simulink model "DemonstratorSimscape_GMM1"  (R2021b)
settings: Solver=ode113  StartTime=0.0  StopTime=t_stop*0+20  FixedStep=1e-4
values from neighbouring files (symbols this model uses):
  brkD = 0    [main.m]
  brkI = 1e4    (= 10000)    [main.m]
  brkP = 1e5    (= 100000)    [main.m]
  d_drm = 0.5*d_drum    [main.m]
  d_shm = 0.4*d_sheave    [main.m]
  DeltaCable0 = 0    [main.m]
  Droop_scaling = 0    [main.m]
  eta_sh = 0.015    [main.m]
  filt_NUM = ones(1,200)*0.005    [main.m]
  g = 9.80665    [main.m]
  Iw = 0.5*(W.i + M.in*GB.r^2)    [main.m]
  Kp_mul = 0.3    [main.m]
  Lc0 = abs((T.ph-L.height-P.d-L.z0)*0.001)    [main.m]
  Ls1 = ((T.ph-0.5*W.pd)/1000)    [main.m]
  Ls2 = ((0.5*(T.s2+P.d)-2*P.d)/1000)    [main.m]
  M = 50e3    (= 50000)    [calcGrav.m]
  phi0_drm = -90    [main.m]
  phi0_shm = -90    [main.m]
  r_sheave = P.d*0.5    [main.m]
  s = tf('s')    [calcGrav.m]
  tau_brk = 0.001    [main.m]
  tau_em = 60e-3    (= 0.06)    [calcGrav.m]    (also in main.m)
  tau_m = tau_w/GB.r    [main.m]
  Tmax = 400e3    (= 400000)    [main.m]
  Tn_mul = 10    [main.m]
  x_drm = 0.7*r_drum    [main.m]
  x_shm = 0.7*r_sheave    [main.m]
  z0 = 0    [calcGrav.m]    (also in main.m = L.z0-P.d*0.5-P.d-P.d-L.height-T.h1-T.h2-32)
undefined symbols (not defined in the file or in its folder): C, CA, Controller_sampleTime, DiscIntNeverNeededParam, GB, L, P, Part, T, VFD_acceleration_model_factor, VFD_Adapt_factor_lower_p1458, VFD_Adapt_factor_upper_p1459, VFD_Curr_limit_var_p0641, VFD_Current_limit_p0640, VFD_Id_setp_total_r1624, VFD_Iq, VFD_Kp_n_basic_p1460, VFD_M, VFD_M_accel_T_smooth_p1517, VFD_M_lim_var_fixS_src_p1551, VFD_M_max_lower_p1521, VFD_M_max_lower_scal_p1525, VFD_M_max_up_mot_scal_p1524, VFD_M_max_upper_p1520, VFD_n_act_T_smooth_p1442, VFD_n_ctr_Kp_n_up_scal_p1461, VFD_n_ctr_Tn_n_up_sca_p1463, VFD_n_ctrl_adapt_Kp_lower_p1456, VFD_n_ctrl_adapt_Kp_upper_p1457, VFD_n_ctrl_Adpt_sig_Kp_p1455, VFD_n_ctrl_Kp_scal_p1466, VFD_n_ctrl_n_lower_p1464, VFD_n_ctrl_n_upper_p1465, VFD_n_ctrl_Tn_n_lower_p1462, VFD_n_limit_neg_p1086, VFD_n_limit_pos_p1083, VFD_n_limit_setp_p1063, VFD_n_max_p1082, VFD_n_set_filt_1_T_p1416, VFD_P_max_gen_p1531, VFD_P_max_mot_p1530, VFD_PU_I_outp_max_r0289, VFD_RFG_ramp_down_time_p1121, VFD_RFG_ramp_up_time_p1120, VFD_RFG_t_RD_scal_p1139, VFD_RFG_t_RU_scal_p1138, VSD, W, X, Y, Z
libraries: sm_lib x248, nesl_utility x128, simulink x49, cstblocks x2, pid_lib x2, slpidlib x2, simulink_extras x2
(part 4 of 11)

== system DemonstratorSimscape_GMM1/EM System/Motor Winch Right/Gearbox ==
  MotTrq : Inport
  MotSpd : Inport  Port=2
  GearBox : Gain  Gain=GB.r
  Gearbox efficiency : Subsystem
  Sheaves efficiency : Subsystem
  WinchTrq : Outport
  WinchTrq' : Outport  Port=2
  wires:
  Gearbox efficiency/1(WinchTrq) -> GearBox/1
  MotTrq/1 -> Gearbox efficiency/1(MotTrqRef)
  MotSpd/1 -> Sheaves efficiency/2(MotSpd), Gearbox efficiency/2(MotSpd)
  GearBox/1 -> WinchTrq/1, Sheaves efficiency/1(WinchTrq)
  Sheaves efficiency/1(WinchTrq') -> WinchTrq'/1

== system DemonstratorSimscape_GMM1/EM System/Motor Winch Right/Motor ==
  MotTrqRef : Inport
  MotSpd : Inport  Port=2
  Ideal motor : Subsystem  Commented=on
  Motor dynamics : Subsystem
  Motor with efficiency : Subsystem
  MotTrq : Outport
  wires:
  MotTrqRef/1 -> Motor with efficiency/1(MotTrqRef), Ideal motor/1(MotTrqRef)
  MotSpd/1 -> Motor with efficiency/2(MotSpd)
  Motor dynamics/1(TrqOut) -> MotTrq/1
  Motor with efficiency/1(MotTrq) -> Motor dynamics/1(TrqIn)

== system DemonstratorSimscape_GMM1/EM System/Motor Winch Right/PS>Sim ==
  Gain{1..4} (4 alike) : Gain
  b (rad/s) : nesl_utility/PS-Simulink Converter  PhysicalDomain=network_engine_domain  SubClassName=ps_output  LeftPortType=input  RightPortType=output  PseudoPeriodic=off  Frequencies=[]  Unit=rad/s  AffineConversion=off
      settings: SourceProductBaseCode=PW,SS
  b (rad/s^2) : nesl_utility/PS-Simulink Converter  PhysicalDomain=network_engine_domain  SubClassName=ps_output  LeftPortType=input  RightPortType=output  PseudoPeriodic=off  Frequencies=[]  Unit=rad/s^2  AffineConversion=off
      settings: SourceProductBaseCode=PW,SS
  fc (N) : nesl_utility/PS-Simulink Converter  PhysicalDomain=network_engine_domain  SubClassName=ps_output  LeftPortType=input  RightPortType=output  PseudoPeriodic=off  Frequencies=[]  Unit=N  AffineConversion=off
      settings: SourceProductBaseCode=PW,SS
  ft (N) : nesl_utility/PS-Simulink Converter  PhysicalDomain=network_engine_domain  SubClassName=ps_output  LeftPortType=input  RightPortType=output  PseudoPeriodic=off  Frequencies=[]  Unit=N  AffineConversion=off
      settings: SourceProductBaseCode=PW,SS
  q (deg) : nesl_utility/PS-Simulink Converter  PhysicalDomain=network_engine_domain  SubClassName=ps_output  LeftPortType=input  RightPortType=output  PseudoPeriodic=off  Frequencies=[]  Unit=deg  AffineConversion=off
      settings: SourceProductBaseCode=PW,SS
  t (Nm) : nesl_utility/PS-Simulink Converter  PhysicalDomain=network_engine_domain  SubClassName=ps_output  LeftPortType=input  RightPortType=output  PseudoPeriodic=off  Frequencies=[]  Unit=N*m  AffineConversion=off
      settings: SourceProductBaseCode=PW,SS
  tc (Nm) : nesl_utility/PS-Simulink Converter  PhysicalDomain=network_engine_domain  SubClassName=ps_output  LeftPortType=input  RightPortType=output  PseudoPeriodic=off  Frequencies=[]  Unit=N*m  AffineConversion=off
      settings: SourceProductBaseCode=PW,SS
  tt (Nm) : nesl_utility/PS-Simulink Converter  PhysicalDomain=network_engine_domain  SubClassName=ps_output  LeftPortType=input  RightPortType=output  PseudoPeriodic=off  Frequencies=[]  Unit=N*m  AffineConversion=off
      settings: SourceProductBaseCode=PW,SS
  w (rpm) : nesl_utility/PS-Simulink Converter  PhysicalDomain=network_engine_domain  SubClassName=ps_output  LeftPortType=input  RightPortType=output  PseudoPeriodic=off  Frequencies=[]  Unit=rpm  AffineConversion=off
      settings: SourceProductBaseCode=PW,SS
  q : PMIOPort  Side=Left
  Conn2 : PMIOPort  Port=2  Side=Left
  Conn3 : PMIOPort  Port=3  Side=Left
  Conn4 : PMIOPort  Port=4  Side=Left
  Conn5 : PMIOPort  Port=5  Side=Left
  Conn6 : PMIOPort  Port=6  Side=Left
  Conn7 : PMIOPort  Port=7  Side=Left
  Conn8 : PMIOPort  Port=8  Side=Left
  Out1 : Outport  VectorParamsAs1DForOutWhenUnconnected=off
  Out2 : Outport  Port=2  VectorParamsAs1DForOutWhenUnconnected=off
  Out3 : Outport  Port=3  VectorParamsAs1DForOutWhenUnconnected=off
  Out4 : Outport  Port=4  VectorParamsAs1DForOutWhenUnconnected=off
  Out5 : Outport  Port=5  VectorParamsAs1DForOutWhenUnconnected=off
  Out6 : Outport  Port=6  VectorParamsAs1DForOutWhenUnconnected=off
  Out7 : Outport  Port=7  VectorParamsAs1DForOutWhenUnconnected=off
  Out8 : Outport  Port=8  VectorParamsAs1DForOutWhenUnconnected=off
  Out9 : Outport  Port=9  VectorParamsAs1DForOutWhenUnconnected=off
  wires:
  q (deg)/1 -> Gain1/1
  w (rpm)/1 -> Gain2/1
  b (rad/s^2)/1 -> Gain3/1
  t (Nm)/1 -> Gain4/1
  fc (N)/1 -> Out5/1
  tc (Nm)/1 -> Out6/1
  ft (N)/1 -> Out7/1
  tt (Nm)/1 -> Out8/1
  Gain1/1 -> Out1/1
  Gain2/1 -> Out2/1
  Gain3/1 -> Out3/1
  Gain4/1 -> Out4/1
  b (rad/s)/1 -> Out9/1
  connections:
  q/RConn1 -- q (deg)/LConn1
  Conn2/RConn1 -- b (rad/s)/LConn1 -- w (rpm)/LConn1
  Conn3/RConn1 -- b (rad/s^2)/LConn1
  Conn4/RConn1 -- t (Nm)/LConn1
  fc (N)/LConn1 -- Conn5/RConn1
  Conn6/RConn1 -- tc (Nm)/LConn1
  ft (N)/LConn1 -- Conn7/RConn1
  Conn8/RConn1 -- tt (Nm)/LConn1

== system DemonstratorSimscape_GMM1/EM System/Winch Left (yellow)/Variable Winch Inertia ==
  WinchAngle (deg) : Inport
  Constant : Constant  Value=W.d/2
  Demux : Demux  Outputs=3
  Gain1 : Gain  Gain=-1
  Gain2 : Gain  Gain=0.5
  S-Function : S-Function  FunctionName=sfun_wcable  Parameters=W.n0,W.perc0,W.dpl,W.alpha_r,CA.mpl,W.d,CA.d  SFunctionDeploymentMode=off  EnableBusSupport=off
  Simulink-PS Converter : nesl_utility/Simulink-PS Converter  PhysicalDomain=network_engine_domain  SubClassName=ps_input  LeftPortType=input  RightPortType=output  PseudoPeriodic=off  Frequencies=[]  NoiseDistribution=none  NoiseParameters=[]  Unit=kg  AffineConversion=on  FilteringAndDerivatives=zero  SimscapeFilterOrder=2  InputFilterTimeConstant=0.001  UdotUserProvided=0
      settings: SourceProductBaseCode=PW,SS
  WinchCable : Scope  Commented=on  NumInputPorts=4
  cable on Winch Variable Mass : sm_lib/Body Elements/Variable Mass/General Variable Mass  VariableInertiaType=PointMass  MassType=TimeVarying  Mass=1  MassUnits=kg  CenterOfMassType=Constant  CenterOfMass=[0 0 0]  CenterOfMassUnits=m  InertiaMatrixType=Constant  MomentsOfInertia=[1 1 1]  MomentsOfInertiaUnits=kg*m^2  ProductsOfInertia=[0 0 0]  ProductsOfInertiaUnits=kg*m^2  GraphicType=None  MarkerShape=Sphere  MarkerSize=10  GraphicVisPropType=SimpleVisualProperties  GraphicDiffuseColor=[0.5 0.5 0.5]  GraphicSpecularColor=[0.5 0.5 0.5 1.0]  GraphicAmbientColor=[0.15 0.15 0.15 1.0]  GraphicEmissiveColor=[0.0 0.0 0.0 1.0]  GraphicShininess=75  GraphicOpacity=1.0
      settings: SourceProductBaseCode=MS
  CableInertia : PMIOPort  Side=Right
  CableLayer : Outport
  WinchRadius (mm) : Outport  Port=2  VectorParamsAs1DForOutWhenUnconnected=off
  wires:
  Demux/1 -> WinchCable/3, Simulink-PS Converter/1
  Gain1/1 -> S-Function/1
  S-Function/1 -> Demux/1
  Demux/2 -> WinchCable/1, CableLayer/1
  WinchAngle (deg)/1 -> Gain1/1
  Demux/3 -> WinchRadius (mm)/1
  [CableMass] -> Gain2/1
  Gain2/1 -> WinchCable/4
  Constant/1 -> WinchCable/2
  connections:
  cable on Winch Variable Mass/RConn1 -- CableInertia/RConn1
  Simulink-PS Converter/RConn1 -- cable on Winch Variable Mass/LConn1

== system DemonstratorSimscape_GMM1/EM System/Winch Left (yellow)/tags ==
  Rigid Transform1 : sm_lib/Frames and Transforms/Rigid Transform  TranslationMethod=Cartesian  TranslationStandardOffset=0  TranslationLengthUnit=mm  TranslationStandardAxis=+Z  TranslationCartesianOffset=[x_drm*cosd(phi0+120), x_drm*sind(phi0+120), s*d_drm]  TranslationROffset=0  TranslationROffsetUnits=m  TranslationZOffset=0  TranslationZOffsetUnits=m  TranslationThetaOffset=0  TranslationThetaOffsetUnits=deg  RotationMethod=None  RotationAngleUnits=deg  RotationStandardAxis=+Z  RotationAngle=0.0  RotationArbitraryAxis=[0 0 1]  FollAlignAxisA=+X  BaseAlignAxisA=+Y  FollAlignAxisB=+Y  BaseAlignAxisB=+Z  RotationSequenceAxes=FollowerAxes  RotationSequence=XYX  RotationSequenceAngles=[0 0 0]  RotationSequenceAnglesUnits=deg  RotationMatrix=[1 0 0; 0 1 0; 0 0 1]
  Rigid Transform2 : sm_lib/Frames and Transforms/Rigid Transform  TranslationMethod=Cartesian  TranslationStandardOffset=0  TranslationLengthUnit=mm  TranslationStandardAxis=+Z  TranslationCartesianOffset=[x_drm*cosd(phi0+0), x_drm*sind(phi0+0), s*d_drm]  TranslationROffset=0  TranslationROffsetUnits=m  TranslationZOffset=0  TranslationZOffsetUnits=m  TranslationThetaOffset=0  TranslationThetaOffsetUnits=deg  RotationMethod=None  RotationAngleUnits=deg  RotationStandardAxis=+Z  RotationAngle=0.0  RotationArbitraryAxis=[0 0 1]  FollAlignAxisA=+X  BaseAlignAxisA=+Y  FollAlignAxisB=+Y  BaseAlignAxisB=+Z  RotationSequenceAxes=FollowerAxes  RotationSequence=XYX  RotationSequenceAngles=[0 0 0]  RotationSequenceAnglesUnits=deg  RotationMatrix=[1 0 0; 0 1 0; 0 0 1]
  Rigid Transform3 : sm_lib/Frames and Transforms/Rigid Transform  TranslationMethod=Cartesian  TranslationStandardOffset=0  TranslationLengthUnit=mm  TranslationStandardAxis=+Z  TranslationCartesianOffset=[x_drm*cosd(phi0-120), x_drm*sind(phi0-120), s*d_drm]  TranslationROffset=0  TranslationROffsetUnits=m  TranslationZOffset=0  TranslationZOffsetUnits=m  TranslationThetaOffset=0  TranslationThetaOffsetUnits=deg  RotationMethod=None  RotationAngleUnits=deg  RotationStandardAxis=+Z  RotationAngle=0.0  RotationArbitraryAxis=[0 0 1]  FollAlignAxisA=+X  BaseAlignAxisA=+Y  FollAlignAxisB=+Y  BaseAlignAxisB=+Z  RotationSequenceAxes=FollowerAxes  RotationSequence=XYX  RotationSequenceAngles=[0 0 0]  RotationSequenceAnglesUnits=deg  RotationMatrix=[1 0 0; 0 1 0; 0 0 1]
  tag1 : sm_lib/Body Elements/Cylindrical Solid  GraphicAmbientColor=[0.15 0.15 0.15 1.0]  BasedOnType=Density  CenterOfMass=[0 0 0]  CenterOfMassUnits=m  GraphicDiffuseColor=c_shm  CylinderLength=d_drm  CylinderLengthUnits=mm  CylinderRadius=r_drm  CylinderRadiusUnits=mm  Density=0  DensityUnits=kg/m^3  DoExposeReferenceFrame=on  GraphicEmissiveColor=[0.0 0.0 0.0 1.0]  ExportEntireGeometry=off  SerializedFrames=<Frames/>  MarkerShape=Frame  MarkerSize=10  GraphicType=FromGeometry  InertiaType=CalculateFromGeometry  Mass=0  MassUnits=kg  MomentsOfInertia=[1 1 1]  MomentsOfInertiaUnits=kg*m^2  GraphicOpacity=1.0  ProductsOfInertia=[0 0 0]  ProductsOfInertiaUnits=kg*m^2  GraphicShininess=10  GraphicSpecularColor=[0.8 0.8 0.8]  GraphicVisPropType=SimpleVisualProperties
  tag2 : sm_lib/Body Elements/Cylindrical Solid  GraphicAmbientColor=[0.15 0.15 0.15 1.0]  BasedOnType=Density  CenterOfMass=[0 0 0]  CenterOfMassUnits=m  GraphicDiffuseColor=c_shm  CylinderLength=d_drm  CylinderLengthUnits=mm  CylinderRadius=r_drm  CylinderRadiusUnits=mm  Density=0  DensityUnits=kg/m^3  DoExposeReferenceFrame=on  GraphicEmissiveColor=[0.0 0.0 0.0 1.0]  ExportEntireGeometry=off  SerializedFrames=<Frames/>  MarkerShape=Frame  MarkerSize=10  GraphicType=FromGeometry  InertiaType=CalculateFromGeometry  Mass=0  MassUnits=kg  MomentsOfInertia=[1 1 1]  MomentsOfInertiaUnits=kg*m^2  GraphicOpacity=1.0  ProductsOfInertia=[0 0 0]  ProductsOfInertiaUnits=kg*m^2  GraphicShininess=10  GraphicSpecularColor=[0.8 0.8 0.8]  GraphicVisPropType=SimpleVisualProperties
  tag3 : sm_lib/Body Elements/Cylindrical Solid  GraphicAmbientColor=[0.15 0.15 0.15 1.0]  BasedOnType=Density  CenterOfMass=[0 0 0]  CenterOfMassUnits=m  GraphicDiffuseColor=c_shm  CylinderLength=d_drm  CylinderLengthUnits=mm  CylinderRadius=r_drm  CylinderRadiusUnits=mm  Density=0  DensityUnits=kg/m^3  DoExposeReferenceFrame=on  GraphicEmissiveColor=[0.0 0.0 0.0 1.0]  ExportEntireGeometry=off  SerializedFrames=<Frames/>  MarkerShape=Frame  MarkerSize=10  GraphicType=FromGeometry  InertiaType=CalculateFromGeometry  Mass=0  MassUnits=kg  MomentsOfInertia=[1 1 1]  MomentsOfInertiaUnits=kg*m^2  GraphicOpacity=1.0  ProductsOfInertia=[0 0 0]  ProductsOfInertiaUnits=kg*m^2  GraphicShininess=10  GraphicSpecularColor=[0.8 0.8 0.8]  GraphicVisPropType=SimpleVisualProperties
  Conn1 : PMIOPort  Side=Left
  connections:
  tag2/RConn1 -- Rigid Transform1/RConn1
  Conn1/RConn1 -- Rigid Transform2/LConn1 -- Rigid Transform1/LConn1 -- Rigid Transform3/LConn1
  Rigid Transform2/RConn1 -- tag1/RConn1
  tag3/RConn1 -- Rigid Transform3/RConn1

== system DemonstratorSimscape_GMM1/EM System/Winch Right (blue)/Variable Winch Inertia ==
  WinchAngle (deg) : Inport
  Demux : Demux  Outputs=3
  S-Function : S-Function  FunctionName=sfun_wcable  Parameters=W.n0,W.perc0,W.dpl,W.alpha_r,CA.mpl,W.d,CA.d  SFunctionDeploymentMode=off  EnableBusSupport=off
  Simulink-PS Converter : nesl_utility/Simulink-PS Converter  PhysicalDomain=network_engine_domain  SubClassName=ps_input  LeftPortType=input  RightPortType=output  PseudoPeriodic=off  Frequencies=[]  NoiseDistribution=none  NoiseParameters=[]  Unit=kg  AffineConversion=on  FilteringAndDerivatives=zero  SimscapeFilterOrder=2  InputFilterTimeConstant=0.001  UdotUserProvided=0
      settings: SourceProductBaseCode=PW,SS
  cable on Winch Variable Mass : sm_lib/Body Elements/Variable Mass/General Variable Mass  VariableInertiaType=PointMass  MassType=TimeVarying  Mass=1  MassUnits=kg  CenterOfMassType=Constant  CenterOfMass=[0 0 0]  CenterOfMassUnits=m  InertiaMatrixType=Constant  MomentsOfInertia=[1 1 1]  MomentsOfInertiaUnits=kg*m^2  ProductsOfInertia=[0 0 0]  ProductsOfInertiaUnits=kg*m^2  GraphicType=None  MarkerShape=Sphere  MarkerSize=10  GraphicVisPropType=SimpleVisualProperties  GraphicDiffuseColor=[0.5 0.5 0.5]  GraphicSpecularColor=[0.5 0.5 0.5 1.0]  GraphicAmbientColor=[0.15 0.15 0.15 1.0]  GraphicEmissiveColor=[0.0 0.0 0.0 1.0]  GraphicShininess=75  GraphicOpacity=1.0
      settings: SourceProductBaseCode=MS
  CableInertia : PMIOPort  Side=Right
  CableLayer : Outport
  WinchRadius (mm) : Outport  Port=2  VectorParamsAs1DForOutWhenUnconnected=off
  wires:
  Demux/1 -> Simulink-PS Converter/1
  WinchAngle (deg)/1 -> S-Function/1
  S-Function/1 -> Demux/1
  Demux/2 -> CableLayer/1
  Demux/3 -> WinchRadius (mm)/1
  connections:
  cable on Winch Variable Mass/RConn1 -- CableInertia/RConn1
  Simulink-PS Converter/RConn1 -- cable on Winch Variable Mass/LConn1

== system DemonstratorSimscape_GMM1/EM System/Winch Right (blue)/tags ==
  Rigid Transform1 : sm_lib/Frames and Transforms/Rigid Transform  TranslationMethod=Cartesian  TranslationStandardOffset=0  TranslationLengthUnit=mm  TranslationStandardAxis=+Z  TranslationCartesianOffset=[x_drm*cosd(phi0+120), x_drm*sind(phi0+120), s*d_drm]  TranslationROffset=0  TranslationROffsetUnits=m  TranslationZOffset=0  TranslationZOffsetUnits=m  TranslationThetaOffset=0  TranslationThetaOffsetUnits=deg  RotationMethod=None  RotationAngleUnits=deg  RotationStandardAxis=+Z  RotationAngle=0.0  RotationArbitraryAxis=[0 0 1]  FollAlignAxisA=+X  BaseAlignAxisA=+Y  FollAlignAxisB=+Y  BaseAlignAxisB=+Z  RotationSequenceAxes=FollowerAxes  RotationSequence=XYX  RotationSequenceAngles=[0 0 0]  RotationSequenceAnglesUnits=deg  RotationMatrix=[1 0 0; 0 1 0; 0 0 1]
  Rigid Transform2 : sm_lib/Frames and Transforms/Rigid Transform  TranslationMethod=Cartesian  TranslationStandardOffset=0  TranslationLengthUnit=mm  TranslationStandardAxis=+Z  TranslationCartesianOffset=[x_drm*cosd(phi0+0), x_drm*sind(phi0+0), s*d_drm]  TranslationROffset=0  TranslationROffsetUnits=m  TranslationZOffset=0  TranslationZOffsetUnits=m  TranslationThetaOffset=0  TranslationThetaOffsetUnits=deg  RotationMethod=None  RotationAngleUnits=deg  RotationStandardAxis=+Z  RotationAngle=0.0  RotationArbitraryAxis=[0 0 1]  FollAlignAxisA=+X  BaseAlignAxisA=+Y  FollAlignAxisB=+Y  BaseAlignAxisB=+Z  RotationSequenceAxes=FollowerAxes  RotationSequence=XYX  RotationSequenceAngles=[0 0 0]  RotationSequenceAnglesUnits=deg  RotationMatrix=[1 0 0; 0 1 0; 0 0 1]
  Rigid Transform3 : sm_lib/Frames and Transforms/Rigid Transform  TranslationMethod=Cartesian  TranslationStandardOffset=0  TranslationLengthUnit=mm  TranslationStandardAxis=+Z  TranslationCartesianOffset=[x_drm*cosd(phi0-120), x_drm*sind(phi0-120), s*d_drm]  TranslationROffset=0  TranslationROffsetUnits=m  TranslationZOffset=0  TranslationZOffsetUnits=m  TranslationThetaOffset=0  TranslationThetaOffsetUnits=deg  RotationMethod=None  RotationAngleUnits=deg  RotationStandardAxis=+Z  RotationAngle=0.0  RotationArbitraryAxis=[0 0 1]  FollAlignAxisA=+X  BaseAlignAxisA=+Y  FollAlignAxisB=+Y  BaseAlignAxisB=+Z  RotationSequenceAxes=FollowerAxes  RotationSequence=XYX  RotationSequenceAngles=[0 0 0]  RotationSequenceAnglesUnits=deg  RotationMatrix=[1 0 0; 0 1 0; 0 0 1]
  tag1 : sm_lib/Body Elements/Cylindrical Solid  GraphicAmbientColor=[0.15 0.15 0.15 1.0]  BasedOnType=Density  CenterOfMass=[0 0 0]  CenterOfMassUnits=m  GraphicDiffuseColor=c_shm  CylinderLength=d_drm  CylinderLengthUnits=mm  CylinderRadius=r_drm  CylinderRadiusUnits=mm  Density=0  DensityUnits=kg/m^3  DoExposeReferenceFrame=on  GraphicEmissiveColor=[0.0 0.0 0.0 1.0]  ExportEntireGeometry=off  SerializedFrames=<Frames/>  MarkerShape=Frame  MarkerSize=10  GraphicType=FromGeometry  InertiaType=CalculateFromGeometry  Mass=0  MassUnits=kg  MomentsOfInertia=[1 1 1]  MomentsOfInertiaUnits=kg*m^2  GraphicOpacity=1.0  ProductsOfInertia=[0 0 0]  ProductsOfInertiaUnits=kg*m^2  GraphicShininess=10  GraphicSpecularColor=[0.8 0.8 0.8]  GraphicVisPropType=SimpleVisualProperties
  tag2 : sm_lib/Body Elements/Cylindrical Solid  GraphicAmbientColor=[0.15 0.15 0.15 1.0]  BasedOnType=Density  CenterOfMass=[0 0 0]  CenterOfMassUnits=m  GraphicDiffuseColor=c_shm  CylinderLength=d_drm  CylinderLengthUnits=mm  CylinderRadius=r_drm  CylinderRadiusUnits=mm  Density=0  DensityUnits=kg/m^3  DoExposeReferenceFrame=on  GraphicEmissiveColor=[0.0 0.0 0.0 1.0]  ExportEntireGeometry=off  SerializedFrames=<Frames/>  MarkerShape=Frame  MarkerSize=10  GraphicType=FromGeometry  InertiaType=CalculateFromGeometry  Mass=0  MassUnits=kg  MomentsOfInertia=[1 1 1]  MomentsOfInertiaUnits=kg*m^2  GraphicOpacity=1.0  ProductsOfInertia=[0 0 0]  ProductsOfInertiaUnits=kg*m^2  GraphicShininess=10  GraphicSpecularColor=[0.8 0.8 0.8]  GraphicVisPropType=SimpleVisualProperties
  tag3 : sm_lib/Body Elements/Cylindrical Solid  GraphicAmbientColor=[0.15 0.15 0.15 1.0]  BasedOnType=Density  CenterOfMass=[0 0 0]  CenterOfMassUnits=m  GraphicDiffuseColor=c_shm  CylinderLength=d_drm  CylinderLengthUnits=mm  CylinderRadius=r_drm  CylinderRadiusUnits=mm  Density=0  DensityUnits=kg/m^3  DoExposeReferenceFrame=on  GraphicEmissiveColor=[0.0 0.0 0.0 1.0]  ExportEntireGeometry=off  SerializedFrames=<Frames/>  MarkerShape=Frame  MarkerSize=10  GraphicType=FromGeometry  InertiaType=CalculateFromGeometry  Mass=0  MassUnits=kg  MomentsOfInertia=[1 1 1]  MomentsOfInertiaUnits=kg*m^2  GraphicOpacity=1.0  ProductsOfInertia=[0 0 0]  ProductsOfInertiaUnits=kg*m^2  GraphicShininess=10  GraphicSpecularColor=[0.8 0.8 0.8]  GraphicVisPropType=SimpleVisualProperties
  Conn1 : PMIOPort  Side=Left
  connections:
  tag2/RConn1 -- Rigid Transform1/RConn1
  Conn1/RConn1 -- Rigid Transform2/LConn1 -- Rigid Transform1/LConn1 -- Rigid Transform3/LConn1
  Rigid Transform2/RConn1 -- tag1/RConn1
  tag3/RConn1 -- Rigid Transform3/RConn1

== system DemonstratorSimscape_GMM1/Transmission System/Anchor and Load/CableFlex_Left ==
  disp [m] : Inport
  FlexDisp : Scope  Commented=on  NumInputPorts=4
  Inertia1 : sm_lib/Body Elements/Inertia  InertiaType=PointMass  Mass=0.00000001  MassUnits=kg  CenterOfMass=[0 0 0]  CenterOfMassUnits=m  MomentsOfInertia=[1 1 1]  MomentsOfInertiaUnits=kg*m^2  ProductsOfInertia=[0 0 0]  ProductsOfInertiaUnits=kg*m^2  GraphicType=None  MarkerShape=Inertia  MarkerSize=20  GraphicVisPropType=SimpleVisualProperties  GraphicDiffuseColor=[0.5 0.5 0.5]  GraphicSpecularColor=[0.5 0.5 0.5 1.0]  GraphicAmbientColor=[0.15 0.15 0.15 1.0]  GraphicEmissiveColor=[0.0 0.0 0.0 1.0]  GraphicShininess=75  GraphicOpacity=1.0
  Inertia2 : sm_lib/Body Elements/Inertia  InertiaType=PointMass  Mass=0.00000001  MassUnits=kg  CenterOfMass=[0 0 0]  CenterOfMassUnits=m  MomentsOfInertia=[1 1 1]  MomentsOfInertiaUnits=kg*m^2  ProductsOfInertia=[0 0 0]  ProductsOfInertiaUnits=kg*m^2  GraphicType=None  MarkerShape=Inertia  MarkerSize=20  GraphicVisPropType=SimpleVisualProperties  GraphicDiffuseColor=[0.5 0.5 0.5]  GraphicSpecularColor=[0.5 0.5 0.5 1.0]  GraphicAmbientColor=[0.15 0.15 0.15 1.0]  GraphicEmissiveColor=[0.0 0.0 0.0 1.0]  GraphicShininess=75  GraphicOpacity=1.0
  Mux : Mux  Commented=on  Inputs=2
  Mux1 : Mux  Commented=on  Inputs=2
  PS-Simulink Converter : nesl_utility/PS-Simulink Converter  Commented=on  PhysicalDomain=network_engine_domain  SubClassName=ps_output  LeftPortType=input  RightPortType=output  PseudoPeriodic=off  Frequencies=[]  Unit=m  AffineConversion=off
      settings: SourceProductBaseCode=PW,SS
  PS-Simulink Converter1 : nesl_utility/PS-Simulink Converter  Commented=on  PhysicalDomain=network_engine_domain  SubClassName=ps_output  LeftPortType=input  RightPortType=output  PseudoPeriodic=off  Frequencies=[]  Unit=m/s  AffineConversion=off
      settings: SourceProductBaseCode=PW,SS
  PS-Simulink Converter2 : nesl_utility/PS-Simulink Converter  Commented=on  PhysicalDomain=network_engine_domain  SubClassName=ps_output  LeftPortType=input  RightPortType=output  PseudoPeriodic=off  Frequencies=[]  Unit=m  AffineConversion=off
      settings: SourceProductBaseCode=PW,SS
  PS-Simulink Converter3 : nesl_utility/PS-Simulink Converter  Commented=on  PhysicalDomain=network_engine_domain  SubClassName=ps_output  LeftPortType=input  RightPortType=output  PseudoPeriodic=off  Frequencies=[]  Unit=m/s  AffineConversion=off
      settings: SourceProductBaseCode=PW,SS
  PS-Simulink Converter4 : nesl_utility/PS-Simulink Converter  Commented=on  PhysicalDomain=network_engine_domain  SubClassName=ps_output  LeftPortType=input  RightPortType=output  PseudoPeriodic=off  Frequencies=[]  Unit=m  AffineConversion=off
      settings: SourceProductBaseCode=PW,SS
  PS-Simulink Converter5 : nesl_utility/PS-Simulink Converter  Commented=on  PhysicalDomain=network_engine_domain  SubClassName=ps_output  LeftPortType=input  RightPortType=output  PseudoPeriodic=off  Frequencies=[]  Unit=m/s  AffineConversion=off
      settings: SourceProductBaseCode=PW,SS
  Prismatic Joint : sm_lib/Joints/Prismatic Joint  JointMode=Normal  SenseConstraintForce=off  SenseConstraintForceX=off  SenseConstraintForceY=off  SenseConstraintForceZ=off  SenseConstraintTorque=off  SenseConstraintTorqueX=off  SenseConstraintTorqueY=off  SenseConstraintTorqueZ=off  SenseTotalForce=off  SenseTotalForceX=off  SenseTotalForceY=off  SenseTotalForceZ=off  SenseTotalTorque=off  SenseTotalTorqueX=off  SenseTotalTorqueY=off  SenseTotalTorqueZ=off  CompositeWrenchDir=FollowerOnBase  CompositeWrenchFrame=BaseFrame  EquilibriumPosition=0  EquilibriumPositionUnits=m  SpringStiffness=0  SpringStiffnessUnits=N/m  DampingCoefficient=0  DampingCoefficientUnits=N/(m/s)  TorqueActuationMode=ComputedTorque  MotionActuationMode=InputMotion  SensePosition=off  SenseVelocity=off  SenseAcceleration=off  SenseTorqueForce=off  SenseLowerLimitTorqueForce=off  SenseUpperLimitTorqueForce=off  LowerLimitSpecify=off  LowerLimitBound=-1  LowerLimitBoundUnits=m  LowerLimitStiffness=1e6  LowerLimitStiffnessUnits=N/m  LowerLimitDamping=1e3  LowerLimitDampingUnits=N/(m/s)  LowerLimitTransitionRegionWidth=1e-4  LowerLimitTransitionRegionWidthUnits=m  UpperLimitSpecify=off  UpperLimitBound=1  UpperLimitBoundUnits=m  UpperLimitStiffness=1e6  UpperLimitStiffnessUnits=N/m  UpperLimitDamping=1e3  UpperLimitDampingUnits=N/(m/s)  UpperLimitTransitionRegionWidth=1e-4  UpperLimitTransitionRegionWidthUnits=m  PositionTargetSpecify=on  PositionTargetPriority=High  PositionTargetValue=DeltaCable0*0  PositionTargetValueUnits=mm  VelocityTargetSpecify=off  VelocityTargetPriority=High  VelocityTargetValue=0  VelocityTargetValueUnits=m/s
  Rigid Transform1 : sm_lib/Frames and Transforms/Rigid Transform  TranslationMethod=None  TranslationStandardOffset=0  TranslationLengthUnit=m  TranslationStandardAxis=+Z  TranslationCartesianOffset=[0 0 0]  TranslationROffset=0  TranslationROffsetUnits=m  TranslationZOffset=0  TranslationZOffsetUnits=m  TranslationThetaOffset=0  TranslationThetaOffsetUnits=deg  RotationMethod=StandardAxis  RotationAngleUnits=deg  RotationStandardAxis=+X  RotationAngle=-90  RotationArbitraryAxis=[0 0 1]  FollAlignAxisA=+X  BaseAlignAxisA=+Y  FollAlignAxisB=+Y  BaseAlignAxisB=+Z  RotationSequenceAxes=FollowerAxes  RotationSequence=XYX  RotationSequenceAngles=[0 0 0]  RotationSequenceAnglesUnits=deg  RotationMatrix=[1 0 0; 0 1 0; 0 0 1]
  Rigid Transform2 : sm_lib/Frames and Transforms/Rigid Transform  TranslationMethod=None  TranslationStandardOffset=0  TranslationLengthUnit=m  TranslationStandardAxis=+Z  TranslationCartesianOffset=[0 0 0]  TranslationROffset=0  TranslationROffsetUnits=m  TranslationZOffset=0  TranslationZOffsetUnits=m  TranslationThetaOffset=0  TranslationThetaOffsetUnits=deg  RotationMethod=StandardAxis  RotationAngleUnits=deg  RotationStandardAxis=+X  RotationAngle=90  RotationArbitraryAxis=[0 0 1]  FollAlignAxisA=+X  BaseAlignAxisA=+Y  FollAlignAxisB=+Y  BaseAlignAxisB=+Z  RotationSequenceAxes=FollowerAxes  RotationSequence=XYX  RotationSequenceAngles=[0 0 0]  RotationSequenceAnglesUnits=deg  RotationMatrix=[1 0 0; 0 1 0; 0 0 1]
  Simulink-PS Converter1 : nesl_utility/Simulink-PS Converter  PhysicalDomain=network_engine_domain  SubClassName=ps_input  LeftPortType=input  RightPortType=output  PseudoPeriodic=off  Frequencies=[]  NoiseDistribution=none  NoiseParameters=[]  Unit=m  AffineConversion=on  FilteringAndDerivatives=filter  SimscapeFilterOrder=2  InputFilterTimeConstant=0.001  UdotUserProvided=2
      settings: SourceProductBaseCode=PW,SS
  Transform Sensor : sm_lib/Frames and Transforms/Transform Sensor  Commented=on  MeasurementFrame=World  SenseAngle=off  SenseAxis=off  SenseAngle1=off  SenseAngle2=off  SenseAngle3=off  SenseQ=off  SenseR=off  SenseOmegaX=off  SenseOmegaY=off  SenseOmegaZ=off  SenseOmega1=off  SenseOmega2=off  SenseOmega3=off  SenseQDot=off  SenseRDot=off  SenseAlphaX=off  SenseAlphaY=off  SenseAlphaZ=off  SenseAlpha1=off  SenseAlpha2=off  SenseAlpha3=off  SenseQDDot=off  SenseRDDot=off  SenseX=off  SenseY=on  SenseZ=off  SenseRad=off  SenseAzim=off  SenseDist=off  SenseInc=off  SenseXDot=off  SenseYDot=on  SenseZDot=off  SenseRadDot=off  SenseAzimDot=off  SenseDistDot=off  SenseIncDot=off  SenseXDDot=off  SenseYDDot=off  SenseZDDot=off  SenseRadDDot=off  SenseAzimDDot=off  SenseDistDDot=off  SenseIncDDot=off
  Transform Sensor1 : sm_lib/Frames and Transforms/Transform Sensor  Commented=on  MeasurementFrame=World  SenseAngle=off  SenseAxis=off  SenseAngle1=off  SenseAngle2=off  SenseAngle3=off  SenseQ=off  SenseR=off  SenseOmegaX=off  SenseOmegaY=off  SenseOmegaZ=off  SenseOmega1=off  SenseOmega2=off  SenseOmega3=off  SenseQDot=off  SenseRDot=off  SenseAlphaX=off  SenseAlphaY=off  SenseAlphaZ=off  SenseAlpha1=off  SenseAlpha2=off  SenseAlpha3=off  SenseQDDot=off  SenseRDDot=off  SenseX=off  SenseY=on  SenseZ=off  SenseRad=off  SenseAzim=off  SenseDist=off  SenseInc=off  SenseXDot=off  SenseYDot=on  SenseZDot=off  SenseRadDot=off  SenseAzimDot=off  SenseDistDot=off  SenseIncDot=off  SenseXDDot=off  SenseYDDot=off  SenseZDDot=off  SenseRadDDot=off  SenseAzimDDot=off  SenseDistDDot=off  SenseIncDDot=off
  Transform Sensor2 : sm_lib/Frames and Transforms/Transform Sensor  Commented=on  MeasurementFrame=World  SenseAngle=off  SenseAxis=off  SenseAngle1=off  SenseAngle2=off  SenseAngle3=off  SenseQ=off  SenseR=off  SenseOmegaX=off  SenseOmegaY=off  SenseOmegaZ=off  SenseOmega1=off  SenseOmega2=off  SenseOmega3=off  SenseQDot=off  SenseRDot=off  SenseAlphaX=off  SenseAlphaY=off  SenseAlphaZ=off  SenseAlpha1=off  SenseAlpha2=off  SenseAlpha3=off  SenseQDDot=off  SenseRDDot=off  SenseX=off  SenseY=on  SenseZ=off  SenseRad=off  SenseAzim=off  SenseDist=off  SenseInc=off  SenseXDot=off  SenseYDot=on  SenseZDot=off  SenseRadDot=off  SenseAzimDot=off  SenseDistDot=off  SenseIncDot=off  SenseXDDot=off  SenseYDDot=off  SenseZDDot=off  SenseRadDDot=off  SenseAzimDDot=off  SenseDistDDot=off  SenseIncDDot=off
  World Frame : sm_lib/Frames and Transforms/World Frame  Commented=on
  F : PMIOPort  Side=Right
  B : PMIOPort  Port=2  Side=Left
  wires:
  disp [m]/1 -> Simulink-PS Converter1/1
  Mux/1 -> FlexDisp/1
  Mux1/1 -> FlexDisp/3
  PS-Simulink Converter4/1 -> FlexDisp/2
  PS-Simulink Converter5/1 -> FlexDisp/4
  PS-Simulink Converter/1 -> Mux/1
  PS-Simulink Converter1/1 -> Mux1/1
  PS-Simulink Converter2/1 -> Mux/2
  PS-Simulink Converter3/1 -> Mux1/2
  connections:
  B/RConn1 -- Transform Sensor2/LConn1 -- Transform Sensor/RConn1 -- Rigid Transform2/LConn1
  Simulink-PS Converter1/RConn1 -- Prismatic Joint/LConn2
  Inertia2/RConn1 -- Prismatic Joint/LConn1 -- Rigid Transform1/LConn1
  Inertia1/RConn1 -- Prismatic Joint/RConn1 -- Rigid Transform2/RConn1
  F/RConn1 -- Transform Sensor2/RConn1 -- Transform Sensor1/RConn1 -- Rigid Transform1/RConn1
  World Frame/RConn1 -- Transform Sensor1/LConn1 -- Transform Sensor/LConn1
  Transform Sensor/RConn2 -- PS-Simulink Converter/LConn1
  Transform Sensor/RConn3 -- PS-Simulink Converter1/LConn1
  Transform Sensor1/RConn2 -- PS-Simulink Converter2/LConn1
  Transform Sensor1/RConn3 -- PS-Simulink Converter3/LConn1
  Transform Sensor2/RConn2 -- PS-Simulink Converter4/LConn1
  Transform Sensor2/RConn3 -- PS-Simulink Converter5/LConn1

== system DemonstratorSimscape_GMM1/Transmission System/Anchor and Load/CableFlex_Right ==
  disp [m] : Inport
  Inertia1 : sm_lib/Body Elements/Inertia  InertiaType=PointMass  Mass=0.00000001  MassUnits=kg  CenterOfMass=[0 0 0]  CenterOfMassUnits=m  MomentsOfInertia=[1 1 1]  MomentsOfInertiaUnits=kg*m^2  ProductsOfInertia=[0 0 0]  ProductsOfInertiaUnits=kg*m^2  GraphicType=None  MarkerShape=Inertia  MarkerSize=20  GraphicVisPropType=SimpleVisualProperties  GraphicDiffuseColor=[0.5 0.5 0.5]  GraphicSpecularColor=[0.5 0.5 0.5 1.0]  GraphicAmbientColor=[0.15 0.15 0.15 1.0]  GraphicEmissiveColor=[0.0 0.0 0.0 1.0]  GraphicShininess=75  GraphicOpacity=1.0
  Inertia2 : sm_lib/Body Elements/Inertia  InertiaType=PointMass  Mass=0.00000001  MassUnits=kg  CenterOfMass=[0 0 0]  CenterOfMassUnits=m  MomentsOfInertia=[1 1 1]  MomentsOfInertiaUnits=kg*m^2  ProductsOfInertia=[0 0 0]  ProductsOfInertiaUnits=kg*m^2  GraphicType=None  MarkerShape=Inertia  MarkerSize=20  GraphicVisPropType=SimpleVisualProperties  GraphicDiffuseColor=[0.5 0.5 0.5]  GraphicSpecularColor=[0.5 0.5 0.5 1.0]  GraphicAmbientColor=[0.15 0.15 0.15 1.0]  GraphicEmissiveColor=[0.0 0.0 0.0 1.0]  GraphicShininess=75  GraphicOpacity=1.0
  Prismatic Joint : sm_lib/Joints/Prismatic Joint  JointMode=Normal  SenseConstraintForce=off  SenseConstraintForceX=off  SenseConstraintForceY=off  SenseConstraintForceZ=off  SenseConstraintTorque=off  SenseConstraintTorqueX=off  SenseConstraintTorqueY=off  SenseConstraintTorqueZ=off  SenseTotalForce=off  SenseTotalForceX=off  SenseTotalForceY=off  SenseTotalForceZ=off  SenseTotalTorque=off  SenseTotalTorqueX=off  SenseTotalTorqueY=off  SenseTotalTorqueZ=off  CompositeWrenchDir=FollowerOnBase  CompositeWrenchFrame=BaseFrame  EquilibriumPosition=0  EquilibriumPositionUnits=m  SpringStiffness=0  SpringStiffnessUnits=N/m  DampingCoefficient=0  DampingCoefficientUnits=N/(m/s)  TorqueActuationMode=ComputedTorque  MotionActuationMode=InputMotion  SensePosition=off  SenseVelocity=off  SenseAcceleration=off  SenseTorqueForce=off  SenseLowerLimitTorqueForce=off  SenseUpperLimitTorqueForce=off  LowerLimitSpecify=off  LowerLimitBound=-1  LowerLimitBoundUnits=m  LowerLimitStiffness=1e6  LowerLimitStiffnessUnits=N/m  LowerLimitDamping=1e3  LowerLimitDampingUnits=N/(m/s)  LowerLimitTransitionRegionWidth=1e-4  LowerLimitTransitionRegionWidthUnits=m  UpperLimitSpecify=off  UpperLimitBound=1  UpperLimitBoundUnits=m  UpperLimitStiffness=1e6  UpperLimitStiffnessUnits=N/m  UpperLimitDamping=1e3  UpperLimitDampingUnits=N/(m/s)  UpperLimitTransitionRegionWidth=1e-4  UpperLimitTransitionRegionWidthUnits=m  PositionTargetSpecify=on  PositionTargetPriority=High  PositionTargetValue=DeltaCable0*0  PositionTargetValueUnits=mm  VelocityTargetSpecify=off  VelocityTargetPriority=High  VelocityTargetValue=0  VelocityTargetValueUnits=m/s
  Rigid Transform1 : sm_lib/Frames and Transforms/Rigid Transform  TranslationMethod=None  TranslationStandardOffset=0  TranslationLengthUnit=m  TranslationStandardAxis=+Z  TranslationCartesianOffset=[0 0 0]  TranslationROffset=0  TranslationROffsetUnits=m  TranslationZOffset=0  TranslationZOffsetUnits=m  TranslationThetaOffset=0  TranslationThetaOffsetUnits=deg  RotationMethod=StandardAxis  RotationAngleUnits=deg  RotationStandardAxis=+X  RotationAngle=-90  RotationArbitraryAxis=[0 0 1]  FollAlignAxisA=+X  BaseAlignAxisA=+Y  FollAlignAxisB=+Y  BaseAlignAxisB=+Z  RotationSequenceAxes=FollowerAxes  RotationSequence=XYX  RotationSequenceAngles=[0 0 0]  RotationSequenceAnglesUnits=deg  RotationMatrix=[1 0 0; 0 1 0; 0 0 1]
  Rigid Transform2 : sm_lib/Frames and Transforms/Rigid Transform  TranslationMethod=None  TranslationStandardOffset=0  TranslationLengthUnit=m  TranslationStandardAxis=+Z  TranslationCartesianOffset=[0 0 0]  TranslationROffset=0  TranslationROffsetUnits=m  TranslationZOffset=0  TranslationZOffsetUnits=m  TranslationThetaOffset=0  TranslationThetaOffsetUnits=deg  RotationMethod=StandardAxis  RotationAngleUnits=deg  RotationStandardAxis=+X  RotationAngle=90  RotationArbitraryAxis=[0 0 1]  FollAlignAxisA=+X  BaseAlignAxisA=+Y  FollAlignAxisB=+Y  BaseAlignAxisB=+Z  RotationSequenceAxes=FollowerAxes  RotationSequence=XYX  RotationSequenceAngles=[0 0 0]  RotationSequenceAnglesUnits=deg  RotationMatrix=[1 0 0; 0 1 0; 0 0 1]
  Simulink-PS Converter1 : nesl_utility/Simulink-PS Converter  PhysicalDomain=network_engine_domain  SubClassName=ps_input  LeftPortType=input  RightPortType=output  PseudoPeriodic=off  Frequencies=[]  NoiseDistribution=none  NoiseParameters=[]  Unit=m  AffineConversion=on  FilteringAndDerivatives=filter  SimscapeFilterOrder=2  InputFilterTimeConstant=0.001  UdotUserProvided=2
      settings: SourceProductBaseCode=PW,SS
  F : PMIOPort  Side=Right
  B : PMIOPort  Port=2  Side=Left
  wires:
  disp [m]/1 -> Simulink-PS Converter1/1
  connections:
  B/RConn1 -- Rigid Transform2/LConn1
  Simulink-PS Converter1/RConn1 -- Prismatic Joint/LConn2
  Inertia2/RConn1 -- Prismatic Joint/LConn1 -- Rigid Transform1/LConn1
  Inertia1/RConn1 -- Prismatic Joint/RConn1 -- Rigid Transform2/RConn1
  F/RConn1 -- Rigid Transform1/RConn1

== system DemonstratorSimscape_GMM1/Transmission System/Anchor and Load/CableRigid_Left ==
  F : PMIOPort  Side=Right
  B : PMIOPort  Port=2  Side=Left
  connections:
  B/RConn1 -- F/RConn1

== system DemonstratorSimscape_GMM1/Transmission System/Anchor and Load/CableRigid_Right ==
  F : PMIOPort  Side=Right
  B : PMIOPort  Port=2  Side=Left
  connections:
  B/RConn1 -- F/RConn1

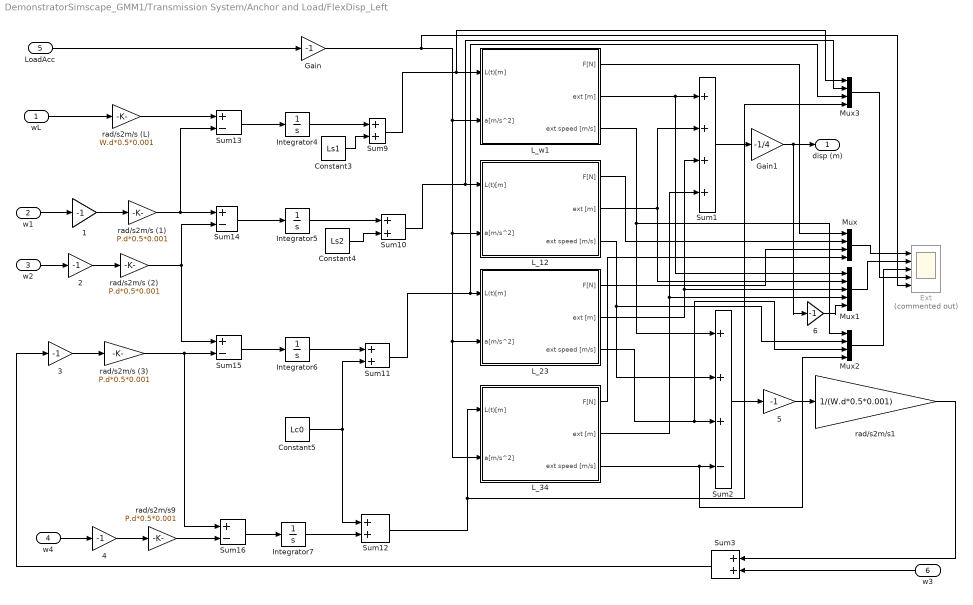
== system DemonstratorSimscape_GMM1/Transmission System/Anchor and Load/FlexDisp_Left ==
  wL : Inport
  w1 : Inport  Port=2
  w2 : Inport  Port=3
  w4 : Inport  Port=4
  LoadAcc : Inport  Port=5
  w3 : Inport  Port=6
  {1..6} (6 alike) : Gain  Gain=-1
  Constant3 : Constant  Value=Ls1
  Constant4 : Constant  Value=Ls2
  Constant5 : Constant  Value=Lc0
  Ext : Scope  Commented=on  NumInputPorts=5
  Gain : Gain  Gain=-1
  Gain1 : Gain  Gain=-1/4
  Integrator{4..7} (4 alike) : Integrator
  L_12 : Subsystem
      settings: MinAlgLoopOccurrences=on
  L_23 : Subsystem
      settings: MinAlgLoopOccurrences=on
  L_34 : Subsystem
      settings: MinAlgLoopOccurrences=on
  L_w1 : Subsystem
      settings: MinAlgLoopOccurrences=on
  Mux : Mux
  Mux1 : Mux  Inputs=5
  Mux2 : Mux
  Mux3 : Mux
  Sum1 : Sum  Inputs=++++
  Sum{3,9..12} (5 alike) : Sum
  Sum{13..16} (4 alike) : Sum  Inputs=+-
  Sum2 : Sum  Inputs=+++-
  rad/s2m/s (1) : Gain  Gain=P.d*0.5*0.001
  rad/s2m/s (2) : Gain  Gain=P.d*0.5*0.001
  rad/s2m/s (3) : Gain  Gain=P.d*0.5*0.001
  rad/s2m/s (L) : Gain  Gain=W.d*0.5*0.001
  rad/s2m/s1 : Gain  Gain=1/(W.d*0.5*0.001)
  rad/s2m/s9 : Gain  Gain=P.d*0.5*0.001
  disp (m) : Outport
  wires:
  wL/1 -> rad/s2m/s (L)/1
  Integrator4/1 -> Sum9/1
  Sum15/1 -> Integrator6/1
  Sum9/1 -> L_w1/1(L(t)[m]), Mux3/1
  rad/s2m/s (1)/1 -> Sum14/1, Sum13/2
  LoadAcc/1 -> Gain/1
  Constant3/1 -> Sum9/2
  Sum12/1 -> L_34/1(L(t)[m]), Mux3/4
  Sum10/1 -> Mux3/2, L_12/1(L(t)[m])
  Integrator5/1 -> Sum10/1
  3/1 -> rad/s2m/s (3)/1
  2/1 -> rad/s2m/s (2)/1
  Sum13/1 -> Integrator4/1
  Constant5/1 -> Sum11/2, Sum12/1
  rad/s2m/s9/1 -> Sum16/2
  rad/s2m/s (L)/1 -> Sum13/1
  Integrator6/1 -> Sum11/1
  rad/s2m/s (3)/1 -> Sum15/2, Sum16/1
  w1/1 -> 1/1
  rad/s2m/s (2)/1 -> Sum14/2, Sum15/1
  4/1 -> rad/s2m/s9/1
  Constant4/1 -> Sum10/2
  Sum16/1 -> Integrator7/1
  w4/1 -> 4/1
  Sum14/1 -> Integrator5/1
  L_w1/2(ext [m]) -> Mux1/1, Sum1/1
  Sum11/1 -> Mux3/3, L_23/1(L(t)[m])
  1/1 -> rad/s2m/s (1)/1
  w2/1 -> 2/1
  Integrator7/1 -> Sum12/2
  Sum1/1 -> Gain1/1
  L_12/2(ext [m]) -> Sum1/2, Mux1/2
  L_23/2(ext [m]) -> Mux1/3, Sum1/3
  L_34/2(ext [m]) -> Mux1/4, Sum1/4
  Sum2/1 -> 5/1
  L_34/3(ext speed [m/s]) -> Mux2/4, Sum2/4
  L_23/3(ext speed [m/s]) -> Mux2/3, Sum2/3
  L_12/3(ext speed [m/s]) -> Mux2/2, Sum2/2
  L_w1/3(ext speed [m/s]) -> Mux2/1, Sum2/1
  5/1 -> rad/s2m/s1/1
  rad/s2m/s1/1 -> Sum3/1
  Sum3/1 -> 3/1
  Gain1/1 -> 6/1, disp (m)/1
  Gain/1 -> Ext/5, L_23/2(a[m/s^2]), L_34/2(a[m/s^2]), L_12/2(a[m/s^2]), L_w1/2(a[m/s^2])
  w3/1 -> Sum3/2
  Mux/1 -> Ext/1
  Mux1/1 -> Ext/2
  Mux2/1 -> Ext/3
  L_w1/1(F[N]) -> Mux/1
  L_12/1(F[N]) -> Mux/2
  L_23/1(F[N]) -> Mux/3
  L_34/1(F[N]) -> Mux/4
  6/1 -> Mux1/5
  Mux3/1 -> Ext/4

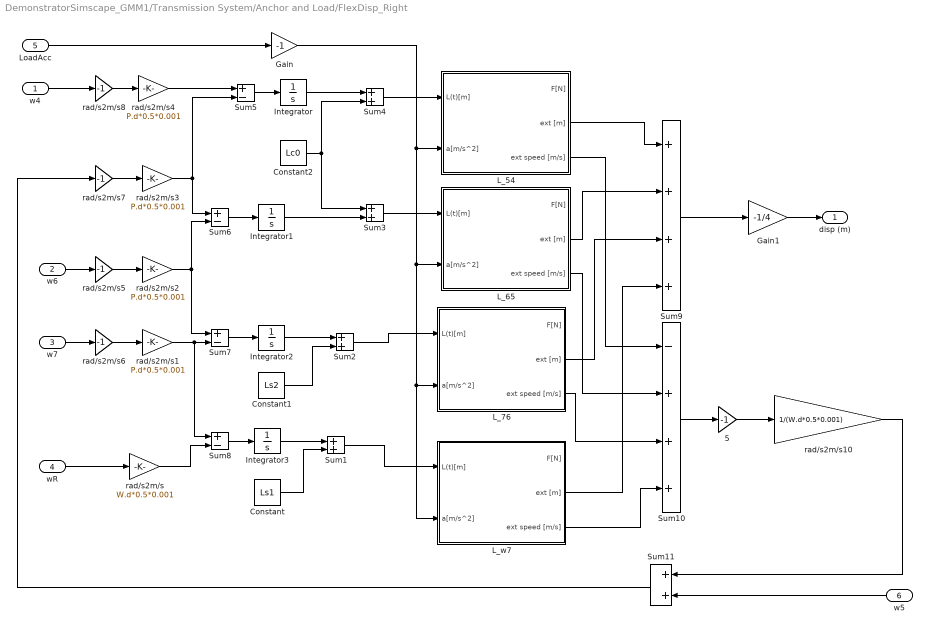
== system DemonstratorSimscape_GMM1/Transmission System/Anchor and Load/FlexDisp_Right ==
  w4 : Inport
  w6 : Inport  Port=2
  w7 : Inport  Port=3
  wR : Inport  Port=4
  LoadAcc : Inport  Port=5
  w5 : Inport  Port=6
  5 : Gain  Gain=-1
  Constant : Constant  Value=Ls1
  Constant1 : Constant  Value=Ls2
  Constant2 : Constant  Value=Lc0
  Gain : Gain  Gain=-1
  Gain1 : Gain  Gain=-1/4
  Integrator{,1..3} (4 alike) : Integrator
  L_54 : Subsystem
      settings: MinAlgLoopOccurrences=on
  L_65 : Subsystem
      settings: MinAlgLoopOccurrences=on
  L_76 : Subsystem
      settings: MinAlgLoopOccurrences=on
  L_w7 : Subsystem
      settings: MinAlgLoopOccurrences=on
  Sum{1..4,11} (5 alike) : Sum
  Sum10 : Sum  Inputs=-+++
  Sum{5..8} (4 alike) : Sum  Inputs=+-
  Sum9 : Sum  Inputs=++++
  rad/s2m/s : Gain  Gain=W.d*0.5*0.001
  rad/s2m/s{1..4} (4 alike) : Gain  Gain=P.d*0.5*0.001
  rad/s2m/s10 : Gain  Gain=1/(W.d*0.5*0.001)
  rad/s2m/s{5..8} (4 alike) : Gain  Gain=-1
  disp (m) : Outport
  wires:
  Sum3/1 -> L_65/1(L(t)[m])
  w6/1 -> rad/s2m/s5/1
  LoadAcc/1 -> Gain/1
  Sum7/1 -> Integrator2/1
  Integrator/1 -> Sum4/1
  Sum4/1 -> L_54/1(L(t)[m])
  rad/s2m/s7/1 -> rad/s2m/s3/1
  rad/s2m/s3/1 -> Sum6/1, Sum5/2
  rad/s2m/s8/1 -> rad/s2m/s4/1
  w4/1 -> rad/s2m/s8/1
  rad/s2m/s6/1 -> rad/s2m/s1/1
  Constant2/1 -> Sum3/1, Sum4/2
  Sum8/1 -> Integrator3/1
  Sum2/1 -> L_76/1(L(t)[m])
  rad/s2m/s/1 -> Sum8/2
  Sum6/1 -> Integrator1/1
  Constant/1 -> Sum1/2
  rad/s2m/s5/1 -> rad/s2m/s2/1
  Sum5/1 -> Integrator/1
  Integrator2/1 -> Sum2/1
  rad/s2m/s2/1 -> Sum6/2, Sum7/1
  Constant1/1 -> Sum2/2
  Integrator1/1 -> Sum3/2
  Sum1/1 -> L_w7/1(L(t)[m])
  rad/s2m/s1/1 -> Sum7/2, Sum8/1
  w7/1 -> rad/s2m/s6/1
  Integrator3/1 -> Sum1/1
  rad/s2m/s4/1 -> Sum5/1
  wR/1 -> rad/s2m/s/1
  Gain/1 -> L_65/2(a[m/s^2]), L_76/2(a[m/s^2]), L_w7/2(a[m/s^2]), L_54/2(a[m/s^2])
  Sum9/1 -> Gain1/1
  L_54/2(ext [m]) -> Sum9/1
  L_65/2(ext [m]) -> Sum9/2
  L_76/2(ext [m]) -> Sum9/3
  L_w7/2(ext [m]) -> Sum9/4
  L_54/3(ext speed [m/s]) -> Sum10/1
  L_65/3(ext speed [m/s]) -> Sum10/2
  L_76/3(ext speed [m/s]) -> Sum10/3
  L_w7/3(ext speed [m/s]) -> Sum10/4
  rad/s2m/s10/1 -> Sum11/1
  Sum10/1 -> 5/1
  5/1 -> rad/s2m/s10/1
  Sum11/1 -> rad/s2m/s7/1
  w5/1 -> Sum11/2
  Gain1/1 -> disp (m)/1

== system DemonstratorSimscape_GMM1/Transmission System/Anchor and Load/Load ==
  CableMass (kg) : Inport
  DOUBLE : Subsystem  Commented=on
  Load Sensors : Subsystem
  Pulley2 Rotation : sm_lib/Frames and Transforms/Rigid Transform  TranslationMethod=None  TranslationStandardOffset=0  TranslationLengthUnit=in  TranslationStandardAxis=+Z  TranslationCartesianOffset=[0 0 0]  TranslationROffset=0  TranslationROffsetUnits=m  TranslationZOffset=0  TranslationZOffsetUnits=m  TranslationThetaOffset=0  TranslationThetaOffsetUnits=deg  RotationMethod=StandardAxis  RotationAngleUnits=deg  RotationStandardAxis=+X  RotationAngle=-90  RotationArbitraryAxis=[0 0 1]  FollAlignAxisA=+Y  BaseAlignAxisA=+Z  FollAlignAxisB=+X  BaseAlignAxisB=+X  RotationSequenceAxes=FollowerAxes  RotationSequence=XYX  RotationSequenceAngles=[0 0 0]  RotationSequenceAnglesUnits=deg  RotationMatrix=[1 0 0; 0 1 0; 0 0 1]
  SINGLE : Subsystem
  F_Left : PMIOPort  Side=Left
  Centre : PMIOPort  Port=2  Side=Right
  F_Right : PMIOPort  Port=3  Side=Left
  LoadAcc (m/s^2) : Outport
  LoadPos (mm) : Outport  Port=2
  LoadVel (m/s) : Outport  Port=3
  wires:
  Load Sensors/2(LoadPos (mm)) -> LoadPos (mm)/1
  CableMass (kg)/1 -> DOUBLE/1(cable mass), SINGLE/1(cable mass)
  Load Sensors/1(LoadAcc (m/s^2)) -> LoadAcc (m/s^2)/1
  Load Sensors/3(LoadVel (m/s)) -> LoadVel (m/s)/1
  connections:
  DOUBLE/RConn2 -- F_Right/RConn1 -- SINGLE/RConn2
  SINGLE/LConn2 -- Load Sensors/RConn1 -- DOUBLE/LConn2
  SINGLE/LConn1 -- DOUBLE/LConn1 -- Pulley2 Rotation/RConn1
  DOUBLE/RConn1 -- SINGLE/RConn1 -- F_Left/RConn1
  Pulley2 Rotation/LConn1 -- Centre/RConn1

== system DemonstratorSimscape_GMM1/Transmission System/Anchor and Load/Sheave_03 ==
  Bending loss : Subsystem  Commented=on
  Gain : Gain  Gain=-1
  Nm : nesl_utility/Simulink-PS Converter  PhysicalDomain=network_engine_domain  SubClassName=ps_input  LeftPortType=input  RightPortType=output  PseudoPeriodic=off  Frequencies=[]  NoiseDistribution=none  NoiseParameters=[]  Unit=1  AffineConversion=off  FilteringAndDerivatives=filter  SimscapeFilterOrder=2  InputFilterTimeConstant=tau_bending  UdotUserProvided=0
      settings: SourceProductBaseCode=PW,SS
  PS>Sim1 : Subsystem
  Pulley 3 : sm_lib/Belts and Cables/Pulley  PitchRadius=P.d*0.5  PitchRadiusUnits=mm  InitialWrapAngleLowerBound=0.0  InitialWrapAngleLowerBoundUnits=deg  SenseWrapAngle=off  SensePulleyAngleA=off  SensePulleyAngleB=off  SenseFleetAngleA=off  SenseFleetAngleB=off
      settings: SourceProductBaseCode=MS
  Revolute Pulley3 : sm_lib/Joints/Revolute Joint  JointMode=Normal  SenseConstraintForce=on  SenseConstraintForceX=off  SenseConstraintForceY=off  SenseConstraintForceZ=off  SenseConstraintTorque=on  SenseConstraintTorqueX=off  SenseConstraintTorqueY=off  SenseConstraintTorqueZ=off  SenseTotalForce=on  SenseTotalForceX=off  SenseTotalForceY=off  SenseTotalForceZ=off  SenseTotalTorque=on  SenseTotalTorqueX=off  SenseTotalTorqueY=off  SenseTotalTorqueZ=off  CompositeWrenchDir=FollowerOnBase  CompositeWrenchFrame=BaseFrame  EquilibriumPosition=0  EquilibriumPositionUnits=deg  SpringStiffness=0  SpringStiffnessUnits=N*m/deg  DampingCoefficient=b_pulley  DampingCoefficientUnits=N*m/(deg/s)  TorqueActuationMode=InputTorque  MotionActuationMode=ComputedMotion  SensePosition=on  SenseVelocity=on  SenseAcceleration=on  SenseTorqueForce=on  SenseLowerLimitTorqueForce=off  SenseUpperLimitTorqueForce=off  LowerLimitSpecify=off  LowerLimitBound=-90  LowerLimitBoundUnits=deg  LowerLimitStiffness=1e4  LowerLimitStiffnessUnits=N*m/deg  LowerLimitDamping=10  LowerLimitDampingUnits=N*m/(deg/s)  LowerLimitTransitionRegionWidth=0.1  LowerLimitTransitionRegionWidthUnits=deg  UpperLimitSpecify=off  UpperLimitBound=90  UpperLimitBoundUnits=deg  UpperLimitStiffness=1e4  UpperLimitStiffnessUnits=N*m/deg  UpperLimitDamping=10  UpperLimitDampingUnits=N*m/(deg/s)  UpperLimitTransitionRegionWidth=0.1  UpperLimitTransitionRegionWidthUnits=deg  PositionTargetSpecify=off  PositionTargetPriority=High  PositionTargetValue=0  PositionTargetValueUnits=deg  VelocityTargetSpecify=off  VelocityTargetPriority=High  VelocityTargetValue=0  VelocityTargetValueUnits=deg/s
  ScopePulley3 : Scope  Commented=on  NumInputPorts=8
  Sheave3 : Subsystem
      mask Display: image('sm_cable_drive_right_angle_pulleyA_IMAGE.png');
  w0 (rad/s) : nesl_utility/PS-Simulink Converter  PhysicalDomain=network_engine_domain  SubClassName=ps_output  LeftPortType=input  RightPortType=output  PseudoPeriodic=off  Frequencies=[]  Unit=rad/s  AffineConversion=on
      settings: SourceProductBaseCode=PW,SS
  WireA : PMIOPort  Side=Left
  ConnS3 : PMIOPort  Port=2  Side=Right
  WireB : PMIOPort  Port=3  Side=Left
  w (rad/s) : Outport
  tag scope: S3=global, w3=global
  wires:
  PS>Sim1/1(Out1) -> ScopePulley3/1
  PS>Sim1/2(Out2) -> ScopePulley3/2
  PS>Sim1/7(Out7) -> ScopePulley3/7
  PS>Sim1/3(Out3) -> ScopePulley3/3
  PS>Sim1/5(Out5) -> ScopePulley3/5
  PS>Sim1/4(Out4) -> ScopePulley3/4
  PS>Sim1/6(Out6) -> ScopePulley3/6
  PS>Sim1/8(Out8) -> ScopePulley3/8
  w0 (rad/s)/1 -> Gain/1, w (rad/s)/1
  [S2] -> Bending loss/1(Sin (kN))
  Bending loss/1(dT (Nm)) -> Nm/1
  Bending loss/2(Sout (kN)) -> [S3]
  Gain/1 -> [w3], Bending loss/2(w (deg/s))
  connections:
  Sheave3/LConn1 -- Revolute Pulley3/RConn1
  Revolute Pulley3/RConn9 -- PS>Sim1/LConn8
  Sheave3/RConn1 -- Pulley 3/LConn1
  WireA/RConn1 -- Pulley 3/RConn1
  Revolute Pulley3/RConn8 -- PS>Sim1/LConn7
  w0 (rad/s)/LConn1 -- Revolute Pulley3/RConn3 -- PS>Sim1/LConn2
  Revolute Pulley3/RConn4 -- PS>Sim1/LConn3
  Revolute Pulley3/RConn7 -- PS>Sim1/LConn6
  Revolute Pulley3/RConn5 -- PS>Sim1/LConn4
  Revolute Pulley3/RConn2 -- PS>Sim1/LConn1
  Revolute Pulley3/LConn1 -- ConnS3/RConn1
  Revolute Pulley3/RConn6 -- PS>Sim1/LConn5
  WireB/RConn1 -- Pulley 3/RConn2
  Nm/RConn1 -- Revolute Pulley3/LConn2
